simulink model "model_new"  (R2021a)
settings: Solver=VariableStepAuto  StartTime=0.0  StopTime=10  FixedStep=0.01  RelTol=1e-3
values from neighbouring files (symbols this model uses):
  b = .071    (= 0.071)    [main.m]
  Ipn = 2    [main.m]
  J = 21890.7e-6    (= 0.0218907)    [main.m]
  K = .573    (= 0.573)    [main.m]
  L = 5.4e-3    (= 0.0054)    [main.m]
  M = 171    [main.m]
  R = 1.45    [main.m]
  Ts = 0.001    [main.m]
  U = 48    [main.m]
undefined symbols (not defined in the file or in its folder): g, I, l, m
libraries: simulink x3, pid_lib x1, spsPWMGeneratorDCDCLib x1, eeQuadratureDecoder x1
settings Model: Creator=artof  LastModifiedBy=artof

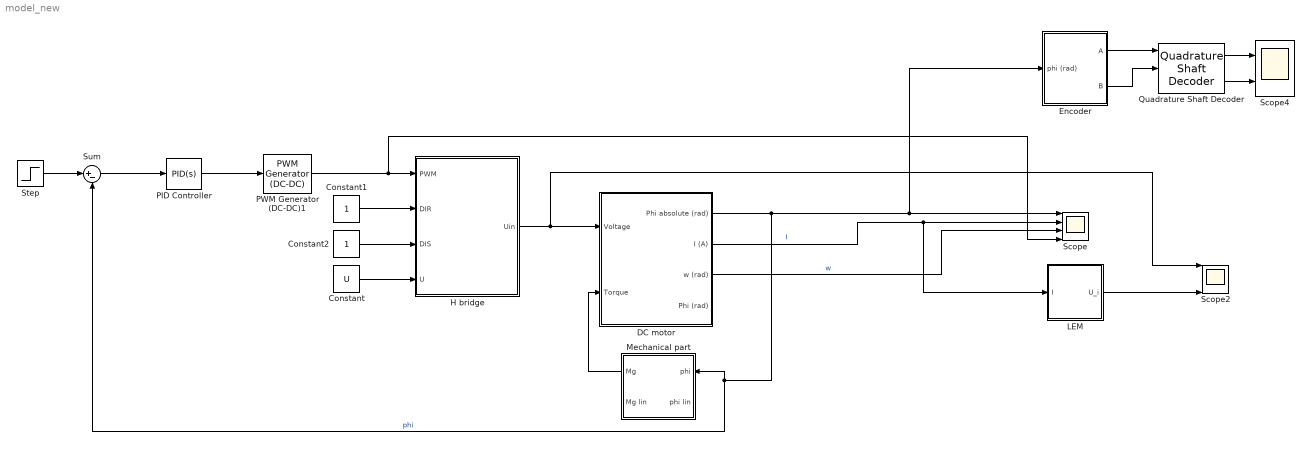
== system model_new ==
  Constant : Constant  Value=U
  Constant1 : Constant
  Constant2 : Constant
  DC motor : Subsystem
  Encoder : Subsystem
  H bridge : Subsystem
  LEM : Subsystem
  Mechanical part : Subsystem
  PID Controller : pid_lib/PID Controller  Controller=PID  Form=Parallel  TimeDomain=Continuous-time  UseExternalTs=off  SampleTime=-1  IntegratorMethod=Forward Euler  FilterMethod=Forward Euler  ControllerParametersSource=internal  P=5  I=5  D=1  UseFilter=on  N=100  TunerSelectOption=Transfer Function Based (PID Tuner App)  InitialConditionSource=internal  InitialConditionForIntegrator=0  InitialConditionForFilter=0  DifferentiatorICPrevScaledInput=0  ExternalReset=none  TrackingMode=off  Kt=1  LimitOutput=off  SatLimitsSource=internal  UpperSaturationLimit=inf  LowerSaturationLimit=-inf  LinearizeAsGain=on  AntiWindupMode=none  Kb=1  POutMin=[]  POutMax=[]  IOutMin=[]  IOutMax=[]  DOutMin=[]  DOutMax=[]  NOutMin=[]  NOutMax=[]  SumOutMin=[]  SumOutMax=[]  SaturationOutMin=[]  SaturationOutMax=[]  PParamMin=[]  PParamMax=[]  IParamMin=[]  IParamMax=[]  DParamMin=[]  DParamMax=[]  NParamMin=[]  NParamMax=[]  KbParamMin=[]  KbParamMax=[]  KtParamMin=[]  KtParamMax=[]  KbOutMin=[]  KbOutMax=[]  KtOutMin=[]  KtOutMax=[]  IntegratorOutMin=[]  IntegratorOutMax=[]  FilterOutMin=[]  FilterOutMax=[]  SumI1OutMin=[]  SumI1OutMax=[]  SumI2OutMin=[]  SumI2OutMax=[]  SumI3OutMin=[]  SumI3OutMax=[]  SumI4OutMin=[]  SumI4OutMax=[]  SumDOutMin=[]  SumDOutMax=[]  DifferentiatorOutMin=[]  DifferentiatorOutMax=[]  FilterDiffOutCoefMin=[]  FilterDiffOutCoefMax=[]  ReciprocalOutMin=[]  ReciprocalOutMax=[]  SumDenOutMin=[]  SumDenOutMax=[]  SumNumOutMin=[]  SumNumOutMax=[]  DivideOutMin=[]  DivideOutMax=[]  UdiffTsProdOutMin=[]  UdiffTsProdOutMax=[]  NTsProdOutMin=[]  NTsProdOutMax=[]  UintegralTsProdOutMin=[]  UintegralTsProdOutMax=[]  UngainTsProdOutMin=[]  UngainTsProdOutMax=[]  IntegratorContinuousStateAttributes=''  IntegratorStateMustResolveToSignalObject=off  IntegratorRTWStateStorageClass=Auto  FilterContinuousStateAttributes=''  FilterStateMustResolveToSignalObject=off  FilterRTWStateStorageClass=Auto  ParallelPVariant=InternalParameters  IdealPVariant=Disabled  IVariant=InternalParameters  DVariant=InternalParameters  IntegratorVariant=Continuous  SatVariant=Disabled  AWVariant=Passthrough  PCopyVariant=Disabled  TRVariant=Disabled  FdbkBlocksVariant=Forward  IdealPFdbkVariant=Disabled  SatFdbkVariant=Disabled  DerivativeFilterVariant=ContFilter  NVariant=InternalParameters  NCopyVariant=Disabled  FilterICVariant=InternalICsFilter  IntegratorICVariant=InternalICs  ExternalResetVariant=Disabled  TRSumVariant=Passthrough  SumFdbkVariant=Disabled  SumVariant=Sum_PID  TsampFilterVariant=InternalTs  TsampNgainVariant=Passthrough  TsampIntegralVariant=Passthrough  ExternalSaturationOutDataTypeStr=Inherit: Same as second input
  PWM Generator (DC-DC)1 : spsPWMGeneratorDCDCLib/PWM Generator (DC-DC)  Fsw=freq  Ts=0
  Quadrature Shaft Decoder : eeQuadratureDecoder/Quadrature Shaft Decoder  NPulse=4  Ts=Ts
      settings: SourceProductBaseCode=PS
  Scope : Scope  NumInputPorts=4
  Scope2 : Scope  NumInputPorts=4
  Scope4 : Scope  NumInputPorts=2
  Step : Step  SampleTime=0
  Sum : Sum  Inputs=|+-
  wires:
  H bridge/1(Uin) -> Scope2/1, DC motor/1("Voltage ")
  DC motor/3(w (rad)) -> Scope/3  "w"
  DC motor/2(I (A)) -> LEM/1(I), Scope/2  "I"
  DC motor/1(Phi absolute (rad)) -> Encoder/1(phi (rad)), Scope/1, Mechanical part/1(phi), Sum/2  "phi"
  Constant2/1 -> H bridge/3(DIS)
  Constant1/1 -> H bridge/2(DIR)
  Constant/1 -> H bridge/4(U)
  PWM Generator (DC-DC)1/1 -> Scope/4, H bridge/1(PWM)
  Sum/1 -> PID Controller/1
  PID Controller/1 -> PWM Generator (DC-DC)1/1
  Mechanical part/1(Mg) -> DC motor/2(Torque)
  Step/1 -> Sum/1
  LEM/1(U_i) -> Scope2/4
  Quadrature Shaft Decoder/1 -> Scope4/1
  Quadrature Shaft Decoder/2 -> Scope4/2
  Encoder/1(A) -> Quadrature Shaft Decoder/1
  Encoder/2(B) -> Quadrature Shaft Decoder/2

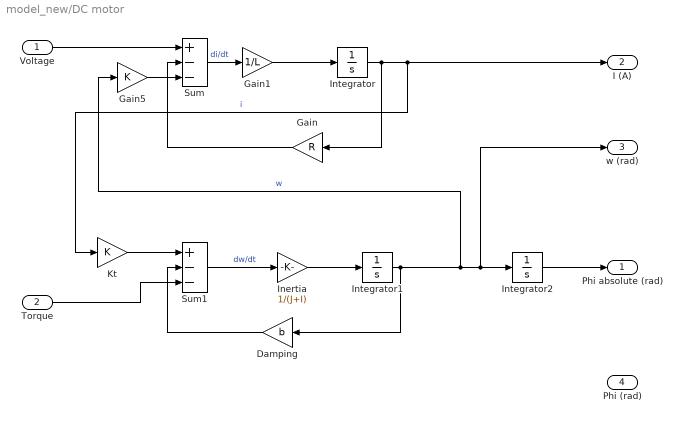
== system model_new/DC motor ==
  "Voltage " : Inport
  Torque : Inport  Port=2
  Damping : Gain  Gain=b
  Gain : Gain  Gain=R
  Gain1 : Gain  Gain=1/L
  Gain5 : Gain  Gain=K
  Inertia : Gain  Gain=1/(J+I)
  Integrator : Integrator
  Integrator1 : Integrator
  Integrator2 : Integrator
  Kt : Gain  Gain=K
  Sum : Sum  Inputs=+--
  Sum1 : Sum  Inputs=+--
  Phi absolute (rad) : Outport
  I (A) : Outport  Port=2
  w (rad) : Outport  Port=3
  Phi (rad) : Outport  Port=4
  wires:
  Gain1/1 -> Integrator/1
  Gain5/1 -> Sum/3
  Inertia/1 -> Integrator1/1
  "Voltage "/1 -> Sum/1
  Integrator/1 -> Gain/1, I (A)/1, Kt/1  "i"
  Integrator1/1 -> Gain5/1, w (rad)/1, Integrator2/1, Damping/1  "w"
  Damping/1 -> Sum1/2
  Sum/1 -> Gain1/1  "di/dt"
  Kt/1 -> Sum1/1
  Gain/1 -> Sum/2
  Sum1/1 -> Inertia/1  "dw/dt"
  Integrator2/1 -> Phi absolute (rad)/1
  Torque/1 -> Sum1/3

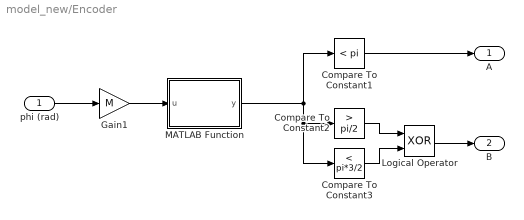
== system model_new/Encoder ==
  phi (rad) : Inport
  Compare To Constant1 : simulink/Logic and Bit Operations/Compare To Constant  relop=<  const=pi  OutDataTypeStr=boolean
  Compare To Constant2 : simulink/Logic and Bit Operations/Compare To Constant  relop=>  const=pi/2  OutDataTypeStr=boolean
  Compare To Constant3 : simulink/Logic and Bit Operations/Compare To Constant  relop=<  const=pi*3/2  OutDataTypeStr=boolean
  Gain1 : Gain  Gain=M
  Logical Operator : Logic  Operator=XOR  AllPortsSameDT=off  OutDataTypeStr=boolean
  MATLAB Function : MATLAB Function  TreatAsAtomicUnit=on
  A : Outport
  B : Outport  Port=2
  wires:
  phi (rad)/1 -> Gain1/1
  Compare To Constant1/1 -> A/1
  Compare To Constant2/1 -> Logical Operator/1
  Logical Operator/1 -> B/1
  Gain1/1 -> MATLAB Function/1(u)
  MATLAB Function/1(y) -> Compare To Constant1/1, Compare To Constant3/1, Compare To Constant2/1
  Compare To Constant3/1 -> Logical Operator/2

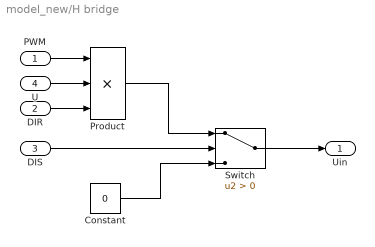
== system model_new/H bridge ==
  PWM : Inport
  DIR : Inport  Port=2
  DIS : Inport  Port=3
  U : Inport  Port=4
  Constant : Constant  Value=0
  Product : Product  Inputs=3
  Switch : Switch  Criteria=u2 > Threshold
  Uin : Outport
  wires:
  U/1 -> Product/2
  PWM/1 -> Product/1
  DIS/1 -> Switch/2
  Constant/1 -> Switch/3
  Switch/1 -> Uin/1
  Product/1 -> Switch/1
  DIR/1 -> Product/3

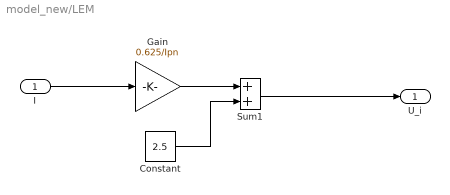
== system model_new/LEM ==
  I : Inport
  Constant : Constant  Value=2.5
  Gain : Gain  Gain=0.625/Ipn
  Sum1 : Sum
  U_i : Outport
  wires:
  Gain/1 -> Sum1/1
  Sum1/1 -> U_i/1
  Constant/1 -> Sum1/2
  I/1 -> Gain/1

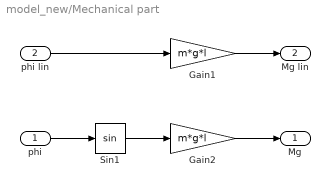
== system model_new/Mechanical part ==
  phi : Inport
  phi lin : Inport  Port=2
  Gain1 : Gain  Gain=m*g*l
  Gain2 : Gain  Gain=m*g*l
  Sin1 : Trigonometry
  Mg : Outport
  Mg lin : Outport  Port=2
  wires:
  Gain2/1 -> Mg/1
  phi/1 -> Sin1/1
  Sin1/1 -> Gain2/1
  Gain1/1 -> Mg lin/1
  phi lin/1 -> Gain1/1

== matlab function model_new/Encoder/MATLAB Function ==
  data: u input; y output
function y = fcn(u)
y = mod(u,2*pi);
